simulink model "prob7"  (R2020b)
settings: Solver=VariableStepAuto  StartTime=0.0  StopTime=10.0  RelTol=1e-3
settings Model: Creator=nadee  LastModifiedBy=nadee

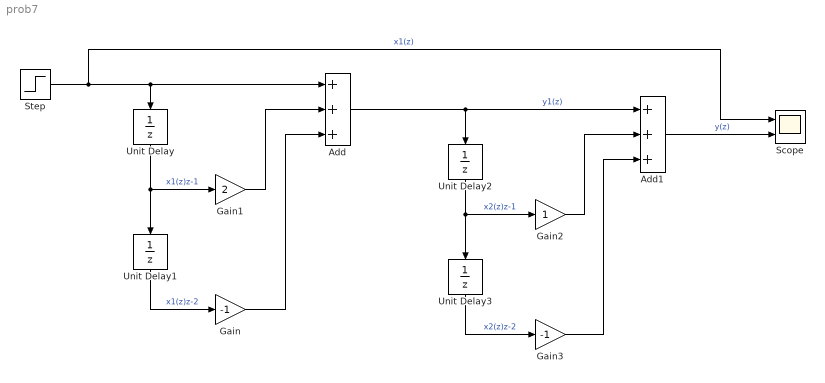
== system prob7 ==
  Add : Sum  Inputs=+++
  Add1 : Sum  Inputs=+++
  Gain : Gain  Gain=-1
  Gain1 : Gain  Gain=2
  Gain2 : Gain
  Gain3 : Gain  Gain=-1
  Scope : Scope  NumInputPorts=2
  Step : Step  SampleTime=0
  Unit Delay{,1..3} (4 alike) : UnitDelay  SampleTime=-1  HasFrameUpgradeWarning=on
  wires:
  Step/1 -> Scope/1, Add/1, Unit Delay/1  "x1(z)"
  Add1/1 -> Scope/2  "y(z)"
  Add/1 -> Unit Delay2/1, Add1/1  "y1(z)"
  Unit Delay/1 -> Gain1/1, Unit Delay1/1  "x1(z)z-1"
  Unit Delay1/1 -> Gain/1  "x1(z)z-2"
  Gain/1 -> Add/3
  Gain1/1 -> Add/2
  Unit Delay2/1 -> Gain2/1, Unit Delay3/1  "x2(z)z-1"
  Unit Delay3/1 -> Gain3/1  "x2(z)z-2"
  Gain3/1 -> Add1/3
  Gain2/1 -> Add1/2
